simulink model "Simulink_resonator"  (R2023a)
settings: Solver=ode4  StartTime=0.0  StopTime=500  FixedStep=0.01  RelTol=1e-3
settings Model: Creator=basti  LastModifiedBy=basti

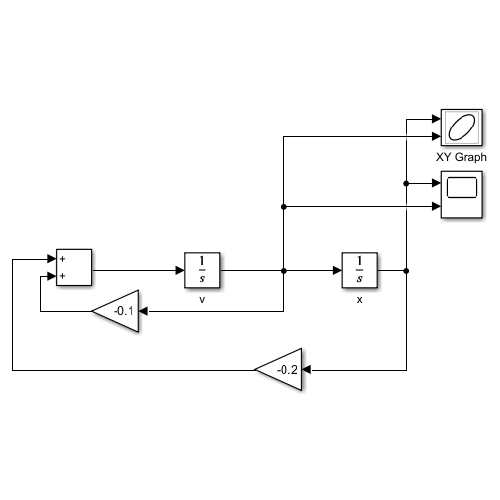
[thumbnail: Simulink's stored preview of the top-level diagram]
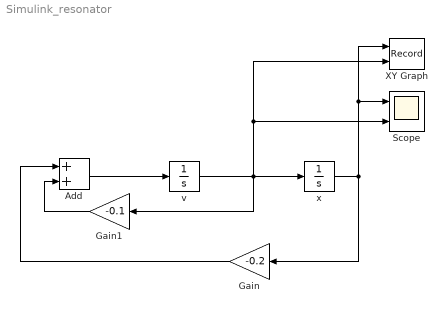
== system Simulink_resonator ==
  Add : Sum
  Gain : Gain  Gain=-0.2
  Gain1 : Gain  Gain=-0.1
  Scope : Scope  NumInputPorts=2
  XY Graph : Record  FileSettingsInternal="{\"entries\":[{\"content\":{\"excelSettings\":{\"content\":{},\"type\":\"Streamout.ExcelSettings\"}},\"type\":\"Streamout.FileSettingStorage\",\"uuid\":\"4ac3fa0b-75e7-4d30-b146-320138278237\"}],\"packageUris\":[\"http://schema.mathworks.com/mf0/streamout_blocks/R2020a\"],\"version\":\"1.0\"}"  Layout=[1 1]  SignalsInternal="{\"entries\":[{\"content\":{\"signals\":[{\"content\":{\"blockPath\":[\"untitled/XY Graph\"],\"dimensions\":[1],\"domain\":\"untitled/XY Graph\",\"lineColor\":\"#a2142f\",\"plots\":[1],\"port\":1,\"sid\":[\"\"],\"signalID\":110,\"signalName\":\"x\"},\"type\":\"RecordBlkView.Signal\",\"uuid\":\"8370f782-c611-4d5c-8764-f0cb00041351\"},{\"content\":{\"blockPath\":[\"untitled/XY Graph\"],\"dimensions\":[1],\"domain\":\"untitled/XY Graph\",\"lineColor\":\"#139fff\",\"plots\":[1],\"port\":2,\"sid\":[\"\"],\"signalID\":114,\"signalName\":\"v\"},\"type\":\"RecordBlkView.Signal\",\"uuid\":\"1b9c63e3-35ff-47eb-aebe-3efdd102feb1\"}]},\"type\":\"RecordBlkView.InputSignals\",\"uuid\":\"4a7aee18-6536-4150-9b75-e088a2aa2e9d\"}],\"packageUris\":[\"http://schema.mathworks.com/mf0/streamout_blocks/R2020a\"],\"version\":\"1.0\"}"  VisualizationBindings="{\"xyplotplugin\":{\"info\":[{\"series\":[{\"bindingParametersList\":[{\"parameter\":\"X-Axis\",\"signalID\":110,\"signalName\":\"x\"},{\"parameter\":\"Y-Axis\",\"signalID\":114,\"signalName\":\"v\"}],\"seriesID\":12401}],\"subplotID\":1}]}}"  CompatibilityTag=XY
  v : Integrator
  x : Integrator  InitialCondition=10
  wires:
  v/1 -> Gain1/1, XY Graph/2, Scope/2, x/1
  x/1 -> XY Graph/1, Scope/1, Gain/1
  Gain/1 -> Add/1
  Gain1/1 -> Add/2
  Add/1 -> v/1
